simulink model "DFIG_BESS_In_power_LFnetwork_5bus"  (R2017b)
settings: Solver=ode23tb  StartTime=0.0  StopTime=7.5  MaxStep=0.04  RelTol=1e-3  EnableMultiTasking=on
values from neighbouring files (symbols this model uses):
  beta = beta (k)    [Parameter_2M_DFIG_BESS.m]
  Cbus = 80e-3    (= 0.08)    [Parameter_2M_DFIG_BESS.m]
  Cbus_bess = 15e-3    (= 0.015)    [Parameter_2M_DFIG_BESS.m]
  Cfilter = 80e-3    (= 0.08)    [Parameter_2M_DFIG_BESS.m]
  cp_opt_abs = abs(max(Cp))    [Parameter_2M_DFIG_BESS.m]
  D = 0.1    [Parameter_2M_DFIG_BESS.m]
  f = 60    [Parameter_2M_DFIG_BESS.m]
  Fs = 1.5    [Parameter_2M_DFIG_BESS.m]
  fsw = 4e3    (= 4000)    [Parameter_2M_DFIG_BESS.m]
  J = 90    [Parameter_2M_DFIG_BESS.m]
  ki_id = (wni^2)*Lr*sigma    (= 491.599501999)    [Parameter_2M_DFIG_BESS.m]
  ki_idg = (wnig^2)*Lg    (= 68.6450725305)    [Parameter_2M_DFIG_BESS.m]
  ki_iq = ki_id    (= 491.599501999)    [Parameter_2M_DFIG_BESS.m]
  ki_iqg = ki_idg    (= 68.6450725305)    [Parameter_2M_DFIG_BESS.m]
  ki_v = -300000    [Parameter_2M_DFIG_BESS.m]
  kp_id = (2*wni*sigma*Lr)-Rr    (= 0.5771)    [Parameter_2M_DFIG_BESS.m]
  kp_idg = (2*wnig*Lg)-Rg    (= 0.364153420404)    [Parameter_2M_DFIG_BESS.m]
  kp_iq = kp_id    (= 0.5771)    [Parameter_2M_DFIG_BESS.m]
  kp_iqg = kp_idg    (= 0.364153420404)    [Parameter_2M_DFIG_BESS.m]
  kp_v = -1000    [Parameter_2M_DFIG_BESS.m]
  Kpg = 1/(1.5*Vs*sqrt(2/3))    [Parameter_2M_DFIG_BESS.m]
  Kqg = -Kpg    [Parameter_2M_DFIG_BESS.m]
  lambda_opt = abs(lambda(posicion))    [Parameter_2M_DFIG_BESS.m]
  Lfilter = 483e-6    (= 0.000483)    [Parameter_2M_DFIG_BESS.m]
  Lg = 483e-6    (= 0.000483)    [Parameter_2M_DFIG_BESS.m]
  Lm = 2.5e-3    (= 0.0025)    [Parameter_2M_DFIG_BESS.m]
  Lr = Lm + Lsr    (= 0.002587)    [Parameter_2M_DFIG_BESS.m]
  Ls = Lm + Lsi    (= 0.002587)    [Parameter_2M_DFIG_BESS.m]
  Lsi = 87e-6    (= 8.7e-05)    [Parameter_2M_DFIG_BESS.m]
  n = 1800    [Parameter_2M_DFIG_BESS.m]
  N = 100    [Parameter_2M_DFIG_BESS.m]
  p = 2    [Parameter_2M_DFIG_BESS.m]
  Ps = 2e6    (= 2000000)    [Parameter_2M_DFIG_BESS.m]
  Radio = 44    [Parameter_2M_DFIG_BESS.m]
  Rfilter = 20e-3    (= 0.02)    [Parameter_2M_DFIG_BESS.m]
  ro = 1.225    [Parameter_2M_DFIG_BESS.m]
  Rr = 2.9e-3    (= 0.0029)    [Parameter_2M_DFIG_BESS.m]
  Rs = 2.6e-3    (= 0.0026)    [Parameter_2M_DFIG_BESS.m]
  sigma = 1- Lm^2/(Ls*Lr)    (= 0.0661284179513)    [Parameter_2M_DFIG_BESS.m]
  Ts = 1/fsw/f    (= 4.16666666667e-06)    [Parameter_2M_DFIG_BESS.m]
  Vbus_ref = 1200    [Parameter_2M_DFIG_BESS.m]
  Vdc_bat_ref = 1300    [Parameter_2M_DFIG_BESS.m]
  Vs = 690    [Parameter_2M_DFIG_BESS.m]
undefined symbols (not defined in the file or in its folder): D1, D11, Delta, DiscIntNeverNeededParam, Ion, Lithium, sigbuilder_block
libraries: powerlib x83, powerlib_meascontrol x28, sps_avr x2, electricdrivelib x1, peGeneralControl x1
(part 1 of 3)
Description:
  | Copyright 2008-2017 The MathWorks, Inc.
settings Model: Creator=MathWorks  LastModifiedBy=admin
settings DataIOCC: LimitDataPoints=on  SaveFormat=Array  SignalLoggingSaveFormat=ModelDataLogs
settings OptimizationCC: ExpressionDepthLimit=2147483647  LifeSpan=inf
settings DebuggingCC: UnderspecifiedInitializationDetection=Classic  MergeDetectMultiDrivingBlocksExec=none  MaxConsecutiveZCsMsg=none  SolverPrmCheckMsg=warning  FcnCallInpInsideContextMsg=warning  UnconnectedInputMsg=none  UnconnectedOutputMsg=none  UnconnectedLineMsg=none  StateNameClashWarn=warning  SFUnexpectedBacktrackingDiag=warning  SFNoUnconditionalDefaultTransitionDiag=warning  SFExecutionAtInitializationDiag=none
settings HardwareCC: ProdBitPerPointer=32  ProdBitPerSizeT=32  ProdBitPerPtrDiffT=32  ProdLargestAtomicFloat=None  ProdIntDivRoundTo=Undefined  ProdEndianess=Unspecified  ProdWordSize=32  ProdHWDeviceType=32-bit Generic
settings ModelReferenceCC: PropagateSignalLabelsOutOfModel=off
settings CodeAppCC: StateflowObjectComments=on
settings GRTTargetCC: TargetLangStandard=C89/C90 (ANSI)  GeneratePreprocessorConditionals=Disable all  CombineOutputUpdateFcns=off  GRTInterface=on
settings ConfigComp: CovMetricSettings=dw  CovHtmlReporting=on  CovSaveCumulativeToWorkspaceVar=on  CovSaveSingleToWorkspaceVar=on  CovExternalEMLEnable=off  CovSFcnEnable=off
settings SimscapeCC: SimscapeNormalizeSystem=off

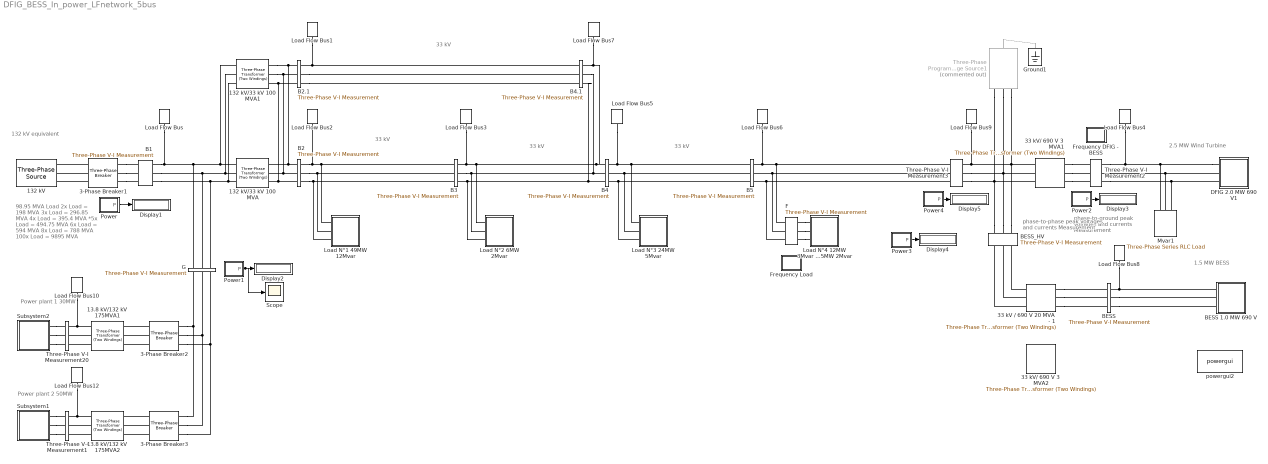
== system DFIG_BESS_In_power_LFnetwork_5bus ==
  note: 98.95 MVA Load
      | 2x Load = 198 MVA
      | 3x Load = 296.85 MVA
      | 4x Load = 395.4 MVA
      | *5x Load = 494.75 MVA
      | 6x Load = 594 MVA
      | 8x Load = 788 MVA
      | 100x Load = 9895 MVA
  note: 2.5 MW Wind Turbine
  note: 33 kV
  note: 132 kV equivalent
  note: 33 kV
  note: 33 kV
  note: phase-to-ground peak voltages
      | and currents Measurement
  note: 33 kV
  note: 1.5 MW BESS
  note: Power plant 1
      | 30MW
  note: Power plant 2
      | 50MW
  note: phase-to-phase peak voltages
      | and currents Measurement
  13.8 kV/132 kV 175MVA1 : powerlib/Elements/Three-Phase Transformer (Two Windings)  Winding1Connection=Delta (D1)  Winding2Connection=Yg  CoreType=Three single-phase transformers  SetSaturation=off  Hysteresis=off  DataFile='basic_model'  SetInitialFlux=off  Measurements=None  UNITS=pu  NominalPower=[100e6 60]  Winding1="[13.8e3  0.002   0.08 ]"  Winding2="[ 132e3  0.002  0.08]"  Rm=500  Lm=500  L0=0.5  Saturation="[ 0,0  ;  0.005,1.2  ;  1.0,1.4 ]"  InitialFluxes=[ 0.8 , -0.8 , 0.7 ]  MoreParameters=off  BreakLoop=off  DataType=off  TransfoNumber=0
  13.8 kV/132 kV 175MVA2 : powerlib/Elements/Three-Phase Transformer (Two Windings)  Winding1Connection=Delta (D1)  Winding2Connection=Yg  CoreType=Three single-phase transformers  SetSaturation=off  Hysteresis=off  DataFile='basic_model'  SetInitialFlux=off  Measurements=None  UNITS=pu  NominalPower=[100e6 60]  Winding1="[13.8e3  0.002   0.08 ]"  Winding2="[ 132e3  0.002  0.08]"  Rm=500  Lm=500  L0=0.5  Saturation="[ 0,0  ;  0.005,1.2  ;  1.0,1.4 ]"  InitialFluxes=[ 0.8 , -0.8 , 0.7 ]  MoreParameters=off  BreakLoop=off  DataType=off  TransfoNumber=0
  132 kV : powerlib/Electrical Sources/Three-Phase Source  InternalConnection=Yg  VoltagePhases=off  Voltage=(132000)  PhaseAngle=-3.3182  Voltage_phases=[25e3 25e3 25e3]/sqrt(3)  PhaseAngles_phases=[0 -120 +120]  Frequency=60  NonIdealSource=on  SpecifyImpedance=on  Resistance=0.8929  Inductance=16.58e-3  ShortCircuitLevel=494e6  BaseVoltage=120e3  XRratio=7  BusType=swing  Pref=10000000  Qref=3000000  Prefabc=[10e3, 10e3, 10e3]  Qrefabc=[0, 0, 0]  Qmin=-Inf  Qmax=Inf
  132 kV/33 kV 100 MVA : powerlib/Elements/Three-Phase Transformer (Two Windings)  Winding1Connection=Yg  Winding2Connection=Delta (D1)  CoreType=Three single-phase transformers  SetSaturation=off  Hysteresis=off  DataFile='basic_model'  SetInitialFlux=off  Measurements=None  UNITS=pu  NominalPower=[100e6 60 ]  Winding1="[ 132e3  0.002    0.06 ]"  Winding2="[ 33e3  0.002  0.06]"  Rm=500  Lm=500  L0=0.5  Saturation="[ 0,0  ;  0.005,1.2  ;  1.0,1.4 ]"  InitialFluxes=[ 0.8 , -0.8 , 0.7 ]  MoreParameters=off  BreakLoop=off  DataType=off  TransfoNumber=0
  132 kV/33 kV 100 MVA1 : powerlib/Elements/Three-Phase Transformer (Two Windings)  Winding1Connection=Yg  Winding2Connection=Delta (D1)  CoreType=Three single-phase transformers  SetSaturation=off  Hysteresis=off  DataFile='basic_model'  SetInitialFlux=off  Measurements=None  UNITS=pu  NominalPower=[100e6 60 ]  Winding1="[ 132e3  0.002    0.06 ]"  Winding2="[ 33e3  0.002  0.06]"  Rm=500  Lm=500  L0=0.5  Saturation="[ 0,0  ;  0.005,1.2  ;  1.0,1.4 ]"  InitialFluxes=[ 0.8 , -0.8 , 0.7 ]  MoreParameters=off  BreakLoop=off  DataType=off  TransfoNumber=0
  3-Phase Breaker1 : powerlib/Elements/Three-Phase Breaker  InitialState=closed  SwitchA=on  SwitchB=on  SwitchC=on  SwitchTimes=[5]  External=off  BreakerResistance=0.001  SnubberResistance=1e6  SnubberCapacitance=inf  Measurements=None
      settings: AttributesFormatString=\n
  3-Phase Breaker2 : powerlib/Elements/Three-Phase Breaker  InitialState=closed  SwitchA=on  SwitchB=on  SwitchC=on  SwitchTimes=[105.025]  External=off  BreakerResistance=0.001  SnubberResistance=1e6  SnubberCapacitance=inf  Measurements=None
      settings: AttributesFormatString=\n
  3-Phase Breaker3 : powerlib/Elements/Three-Phase Breaker  InitialState=closed  SwitchA=on  SwitchB=on  SwitchC=on  SwitchTimes=[105.0]  External=off  BreakerResistance=0.001  SnubberResistance=1e6  SnubberCapacitance=inf  Measurements=None
      settings: AttributesFormatString=\n
  33 kV / 690 V 20 MVA - 1 : powerlib/Elements/Three-Phase Transformer (Two Windings)  Winding1Connection=Delta (D11)  Winding2Connection=Yg  CoreType=Three single-phase transformers  SetSaturation=off  Hysteresis=off  DataFile='hysteresis'  SetInitialFlux=off  Measurements=None  UNITS=SI  NominalPower="[2e6  f]"  Winding1=[33000 0.14881 0.011842]  Winding2=[690 200e-3 2.0881e-06]  Rm=89286  Lm=Inf  L0=0.5  Saturation=[0 0;0.47518 112.54;197.99 142.55]  InitialFluxes=[75.026 -75.026 65.648]  MoreParameters=off  BreakLoop=off  DataType=on  TransfoNumber=0
  33 kV/ 690 V 3 MVA1 : powerlib/Elements/Three-Phase Transformer (Two Windings)  Winding1Connection=Yg  Winding2Connection=Yg  CoreType=Three single-phase transformers  SetSaturation=off  Hysteresis=off  DataFile='hysteresis'  SetInitialFlux=off  Measurements=None  UNITS=pu  NominalPower="[3e6  f]"  Winding1=[33e3 , 0.025/30 , 0.025]  Winding2=[ 690, 0.025/30 , 0.025]  Rm=89286  Lm=inf  L0=0.5  Saturation=[ 0,0 ; 0.0024,1.2 ; 1.0,1.52 ]  InitialFluxes=[ 0.8 , -0.8 , 0.7 ]  MoreParameters=off  BreakLoop=off  DataType=off  TransfoNumber=0
  33 kV/ 690 V 3 MVA2 : powerlib/Elements/Three-Phase Transformer (Two Windings)  Winding1Connection=Yg  Winding2Connection=Yg  CoreType=Three single-phase transformers  SetSaturation=off  Hysteresis=off  DataFile='hysteresis'  SetInitialFlux=off  Measurements=None  UNITS=pu  NominalPower="[2e6  f]"  Winding1=[33e3 , 0.025/30 , 0.025]  Winding2=[ 690, 0.025/30 , 0.025]  Rm=89286  Lm=inf  L0=0.5  Saturation=[ 0,0 ; 0.0024,1.2 ; 1.0,1.52 ]  InitialFluxes=[ 0.8 , -0.8 , 0.7 ]  MoreParameters=off  BreakLoop=off  DataType=off  TransfoNumber=0
  B1 : powerlib/Measurements/Three-Phase V-I Measurement  VoltageMeasurement=phase-to-phase  SetLabelV=on  LabelV=Vabc_B1  Vpu=off  VpuLL=off  CurrentMeasurement=yes  SetLabelI=on  LabelI=Iabc_B1  Ipu=off  Pbase=100e6  Vbase=132e3  OutputType=Complex  PhasorSimulation=off  PSBequivalent=0
  B2 : powerlib/Measurements/Three-Phase V-I Measurement  VoltageMeasurement=no  SetLabelV=off  LabelV=Vabc_B2  Vpu=off  VpuLL=off  CurrentMeasurement=no  SetLabelI=on  LabelI=Iabc_B120  Ipu=off  Pbase=100e6  Vbase=33e3  OutputType=Complex  PhasorSimulation=off  PSBequivalent=0
  B2.1 : powerlib/Measurements/Three-Phase V-I Measurement  VoltageMeasurement=no  SetLabelV=on  LabelV=Vabc_B2  Vpu=on  VpuLL=off  CurrentMeasurement=no  SetLabelI=on  LabelI=Iabc_B120  Ipu=off  Pbase=100e6  Vbase=33e3  OutputType=Complex  PhasorSimulation=off  PSBequivalent=0
  B3 : powerlib/Measurements/Three-Phase V-I Measurement  VoltageMeasurement=no  SetLabelV=on  LabelV=Vabc_B3  Vpu=on  VpuLL=off  CurrentMeasurement=no  SetLabelI=on  LabelI=Iabc_B120  Ipu=off  Pbase=100e6  Vbase=33e3  OutputType=Complex  PhasorSimulation=off  PSBequivalent=0
  B4 : powerlib/Measurements/Three-Phase V-I Measurement  VoltageMeasurement=no  SetLabelV=on  LabelV=Vabc_B4  Vpu=on  VpuLL=off  CurrentMeasurement=no  SetLabelI=on  LabelI=Iabc_B120  Ipu=off  Pbase=100e6  Vbase=33e3  OutputType=Complex  PhasorSimulation=off  PSBequivalent=0
  B4.1 : powerlib/Measurements/Three-Phase V-I Measurement  VoltageMeasurement=no  SetLabelV=on  LabelV=Vabc_B4  Vpu=on  VpuLL=off  CurrentMeasurement=no  SetLabelI=on  LabelI=Iabc_B120  Ipu=off  Pbase=100e6  Vbase=33e3  OutputType=Complex  PhasorSimulation=off  PSBequivalent=0
  B5 : powerlib/Measurements/Three-Phase V-I Measurement  VoltageMeasurement=no  SetLabelV=on  LabelV=Vabc_B5  Vpu=on  VpuLL=off  CurrentMeasurement=no  SetLabelI=on  LabelI=Iabc_B120  Ipu=off  Pbase=100e6  Vbase=33e3  OutputType=Complex  PhasorSimulation=off  PSBequivalent=0
  BESS : powerlib/Measurements/Three-Phase V-I Measurement  VoltageMeasurement=phase-to-phase  SetLabelV=on  LabelV=V_ac_bat_low  Vpu=off  VpuLL=off  CurrentMeasurement=yes  SetLabelI=on  LabelI=I_ac_bat_low  Ipu=off  Pbase=100e6  Vbase=500e3  OutputType=Complex  PhasorSimulation=off  PSBequivalent=0
  BESS 1.0 MW 690 V : Subsystem
  BESS_HV : powerlib/Measurements/Three-Phase V-I Measurement  VoltageMeasurement=phase-to-phase  SetLabelV=on  LabelV=V_ac_bess_HV  Vpu=off  VpuLL=off  CurrentMeasurement=yes  SetLabelI=on  LabelI=I_ac_bess_HV  Ipu=off  Pbase=100e6  Vbase=500e3  OutputType=Complex  PhasorSimulation=off  PSBequivalent=0
  DFIG 2.0 MW 690 V1 : Subsystem
  Display{1..5} (5 alike) : Display
  F : powerlib/Measurements/Three-Phase V-I Measurement  VoltageMeasurement=phase-to-ground  SetLabelV=on  LabelV=Vabc_h_plant  Vpu=off  VpuLL=off  CurrentMeasurement=no  SetLabelI=on  LabelI=Iabc_B120  Ipu=off  Pbase=100e6  Vbase=120e3  OutputType=Complex  PhasorSimulation=off  PSBequivalent=0
  Frequency Load : Subsystem
  Frequency DFIG - BESS : Subsystem
  G : powerlib/Measurements/Three-Phase V-I Measurement  VoltageMeasurement=phase-to-phase  SetLabelV=on  LabelV=Vabc_G  Vpu=off  VpuLL=off  CurrentMeasurement=yes  SetLabelI=on  LabelI=Iabc_G  Ipu=off  Pbase=100e6  Vbase=132e3  OutputType=Complex  PhasorSimulation=off  PSBequivalent=0
  Ground1 : powerlib/Elements/Ground  LConnTagsString=a
  Load Flow Bus : powerlib/Measurements/Load Flow Bus  LConnTagsString=a  Phases=single  Connectors=on one side  ID=B1  Vbase=132e3  Vref=1.02  Vangle=0  VLF=1.02  VLFb=1  VLFc=1  angleLF=0  angleLFb=0  angleLFc=0
      settings: AttributesFormatString=%<ID>\n%<Vbase>V\n%<VLF>pu\n%<angleLF>deg.  SourceProductName=Simscape Power Systems
  Load Flow Bus1 : powerlib/Measurements/Load Flow Bus  LConnTagsString=a  Phases=single  Connectors=on one side  ID=B2.1  Vbase=33e3  Vref=1  Vangle=0  VLF=0.9983  VLFb=1  VLFc=1  angleLF=-30.23  angleLFb=0  angleLFc=0
      settings: AttributesFormatString=%<ID>\n%<Vbase>V\n%<VLF>pu\n%<angleLF>deg.  SourceProductName=Simscape Power Systems
  Load Flow Bus10 : powerlib/Measurements/Load Flow Bus  LConnTagsString=a  Phases=single  Connectors=on one side  ID=B13.8  Vbase=13.8e3  Vref=0.98  Vangle=0  VLF=0.98  VLFb=1  VLFc=1  angleLF=-23.81  angleLFb=0  angleLFc=0
      settings: AttributesFormatString=%<ID>\n%<Vbase>V\n%<VLF>pu\n%<angleLF>deg.  SourceProductName=Simscape Power Systems
  Load Flow Bus12 : powerlib/Measurements/Load Flow Bus  LConnTagsString=a  Phases=single  Connectors=on one side  ID=B13.8  Vbase=13.8e3  Vref=0.98  Vangle=0  VLF=0.98  VLFb=1  VLFc=1  angleLF=-23.81  angleLFb=0  angleLFc=0
      settings: AttributesFormatString=%<ID>\n%<Vbase>V\n%<VLF>pu\n%<angleLF>deg.  SourceProductName=Simscape Power Systems
  Load Flow Bus2 : powerlib/Measurements/Load Flow Bus  LConnTagsString=a  Phases=single  Connectors=on one side  ID=B2  Vbase=33e3  Vref=1  Vangle=0  VLF=0.9983  VLFb=1  VLFc=1  angleLF=-30.23  angleLFb=0  angleLFc=0
      settings: AttributesFormatString=%<ID>\n%<Vbase>V\n%<VLF>pu\n%<angleLF>deg.  SourceProductName=Simscape Power Systems
  Load Flow Bus3 : powerlib/Measurements/Load Flow Bus  LConnTagsString=a  Phases=single  Connectors=on one side  ID=B3  Vbase=33e3  Vref=1  Vangle=0  VLF=0.9671  VLFb=1  VLFc=1  angleLF=-20.87  angleLFb=0  angleLFc=0
      settings: AttributesFormatString=%<ID>\n%<Vbase>V\n%<VLF>pu\n%<angleLF>deg.  SourceProductName=Simscape Power Systems
  Load Flow Bus4 : powerlib/Measurements/Load Flow Bus  LConnTagsString=a  Phases=single  Connectors=on one side  ID=B690  Vbase=690  Vref=1  Vangle=0  VLF=0.9532  VLFb=1  VLFc=1  angleLF=-18.54  angleLFb=0  angleLFc=0
      settings: AttributesFormatString=%<ID>\n%<Vbase>V\n%<VLF>pu\n%<angleLF>deg.  SourceProductName=Simscape Power Systems
  Load Flow Bus5 : powerlib/Measurements/Load Flow Bus  LConnTagsString=a  Phases=single  Connectors=on one side  ID=B4  Vbase=33e3  Vref=1  Vangle=0  VLF=0.9671  VLFb=1  VLFc=1  angleLF=-20.87  angleLFb=0  angleLFc=0
      settings: AttributesFormatString=%<ID>\n%<Vbase>V\n%<VLF>pu\n%<angleLF>deg.  SourceProductName=Simscape Power Systems
  Load Flow Bus6 : powerlib/Measurements/Load Flow Bus  LConnTagsString=a  Phases=single  Connectors=on one side  ID=B5  Vbase=33e3  Vref=1  Vangle=0  VLF=0.9671  VLFb=1  VLFc=1  angleLF=-20.87  angleLFb=0  angleLFc=0
      settings: AttributesFormatString=%<ID>\n%<Vbase>V\n%<VLF>pu\n%<angleLF>deg.  SourceProductName=Simscape Power Systems
  Load Flow Bus7 : powerlib/Measurements/Load Flow Bus  LConnTagsString=a  Phases=single  Connectors=on one side  ID=B4.1  Vbase=33e3  Vref=1  Vangle=0  VLF=0.9671  VLFb=1  VLFc=1  angleLF=-20.87  angleLFb=0  angleLFc=0
      settings: AttributesFormatString=%<ID>\n%<Vbase>V\n%<VLF>pu\n%<angleLF>deg.  SourceProductName=Simscape Power Systems
  Load Flow Bus8 : powerlib/Measurements/Load Flow Bus  LConnTagsString=a  Phases=single  Connectors=on one side  ID=B690_BESS  Vbase=690  Vref=1  Vangle=0  VLF=0.9532  VLFb=1  VLFc=1  angleLF=-18.54  angleLFb=0  angleLFc=0
      settings: AttributesFormatString=%<ID>\n%<Vbase>V\n%<VLF>pu\n%<angleLF>deg.  SourceProductName=Simscape Power Systems
  Load Flow Bus9 : powerlib/Measurements/Load Flow Bus  LConnTagsString=a  Phases=single  Connectors=on one side  ID=B6  Vbase=33e3  Vref=1  Vangle=0  VLF=0.9671  VLFb=1  VLFc=1  angleLF=-20.87  angleLFb=0  angleLFc=0
      settings: AttributesFormatString=%<ID>\n%<Vbase>V\n%<VLF>pu\n%<angleLF>deg.  SourceProductName=Simscape Power Systems
  Load N°1 49MW 12Mvar : Subsystem
  Load N°2 6MW 2Mvar : Subsystem
  Load N°3 24MW 5Mvar : Subsystem
  Load N°4 12MW 3Mvar Load N°5 5MW 2Mvar : Subsystem
  Mvar1 : powerlib/Elements/Three-Phase Series RLC Load  LConnTagsString=A|B|C  Configuration=Delta  NominalVoltage=575  Vabc=[1e3 1e3 1e3]  Vabcp=[1e3 1e3 1e3]  NominalFrequency=60  UnbalancedPower=off  ActivePower=0.05e6/50  InductivePower=0  CapacitivePower=0.05e6  Pabc=[10e3 9e3 11e3]  QLabc=[100 90 110]  QCabc=[100 90 110]  Pabcp=[10e3 9e3 11e3]  QLabcp=[100 90 110]  QCabcp=[100 90 110]  Measurements=None  LoadType=constant Z
  Power : Subsystem
  Power1 : Subsystem
  Power2 : Subsystem
  Power3 : Subsystem
  Power4 : Subsystem
  Scope : Scope
  Subsystem1 : Subsystem
  Subsystem2 : Subsystem
  Three-Phase Programmable Voltage Source1 : powerlib/Electrical Sources/Three-Phase Programmable Voltage Source  Commented=on  PositiveSequence="[33e3  0 f]"  VariationEntity=None  VariationType=Table of time-amplitude pairs  VariationTypeAlt=Step  VariationStep=[-0.5]  VariationRate=-0.3  VariationMagnitude=0.3  VariationFrequency=2  VariationTiming=[5 7.5]  VariationPhaseA=off  Amplitudes=[1 0.95 1]  TimeValues=[0 0.9 2]  HarmonicGeneration=off  HarmonicA=[3 0.2 -25 0]  HarmonicB=[2 0.15 35 2]  Timing="[0.05  3]"  BusType=swing  Pref=0  Qref=0  Qmin=-inf  Qmax=inf
  Three-Phase V-I Measurement1 : powerlib/Measurements/Three-Phase V-I Measurement  VoltageMeasurement=no  SetLabelV=off  LabelV=V_ac_syn_low_2  Vpu=off  VpuLL=off  CurrentMeasurement=no  SetLabelI=off  LabelI=I_ac_syn_low_2  Ipu=off  Pbase=100e6  Vbase=500e3  OutputType=Complex  PhasorSimulation=off  PSBequivalent=0
  Three-Phase V-I Measurement2 : powerlib/Measurements/Three-Phase V-I Measurement  VoltageMeasurement=phase-to-ground  SetLabelV=on  LabelV=V_ac_g  Vpu=off  VpuLL=off  CurrentMeasurement=yes  SetLabelI=on  LabelI=I_ac_g  Ipu=off  Pbase=100e6  Vbase=500e3  OutputType=Complex  PhasorSimulation=off  PSBequivalent=0
  Three-Phase V-I Measurement20 : powerlib/Measurements/Three-Phase V-I Measurement  VoltageMeasurement=no  SetLabelV=on  LabelV=V_ac_syn_low  Vpu=off  VpuLL=off  CurrentMeasurement=no  SetLabelI=on  LabelI=I_ac_syn_low  Ipu=off  Pbase=100e6  Vbase=500e3  OutputType=Complex  PhasorSimulation=off  PSBequivalent=0
  Three-Phase V-I Measurement3 : powerlib/Measurements/Three-Phase V-I Measurement  VoltageMeasurement=phase-to-ground  SetLabelV=on  LabelV=V_ac_g_Total  Vpu=off  VpuLL=off  CurrentMeasurement=yes  SetLabelI=on  LabelI=I_ac_g_Total  Ipu=off  Pbase=100e6  Vbase=500e3  OutputType=Complex  PhasorSimulation=off  PSBequivalent=0
  powergui2 : powerlib/powergui  Priority=1  SimulationMode=Discrete  SampleTime=Ts  frequency=60  Iterations=50  frequencyindice=0  Pbase=100e6  ErrMax=0.0001  UnitsV=kV  UnitsW=MW  buscounter=0  FunctionMessages=off  echomessages=off  EnableUseOfTLC=off  CurrentSourceSwitches=off  DisableSnubberDevices=off  DisableRonSwitches=off  DisableVfSwitches=off  DisplayEquations=off  SolverType=Tustin  Interpol=off  ExternalGateDelay=off  methode=off  Ts=100  x0status=blocks  SPID=off  SwTol=0  HookPort=off  RestoreLinks=warning  ResistiveCurrentMeasurement=off  Frange=[0:2:500]  Ylog=off  Xlog=on  ShowGrid=off  save=off  variable=ZData  structure=0  ZoomFFT=off  StartTime=0.0  cycles=1  DisplayStyle=1  fundamental=60  FreqAxis=off  MaxFrequency=1000  frequencyindicesteady=1  RmsSteady=1  display=off
  wires:
  Power/1(P) -> Display1/1
  Power1/1(P) -> Scope/1, Display2/1
  Power3/1(P) -> Display4/1
  Power2/1(P) -> Display3/1
  Power4/1(P) -> Display5/1
  connections:
  B2/LConn2 -- B2.1/LConn2 -- 132 kV/33 kV 100 MVA1/RConn2 -- 132 kV/33 kV 100 MVA/RConn2
  B2/LConn3 -- B2.1/LConn3 -- 132 kV/33 kV 100 MVA1/RConn3 -- 132 kV/33 kV 100 MVA/RConn3
  B1/RConn1 -- Load Flow Bus/LConn1 -- G/RConn1 -- 132 kV/33 kV 100 MVA1/LConn1 -- 132 kV/33 kV 100 MVA/LConn1
  B2/RConn3 -- B3/LConn3 -- Load N°1 49MW 12Mvar/RConn3
  Load Flow Bus2/LConn1 -- B2/RConn1 -- B3/LConn1 -- Load N°1 49MW 12Mvar/RConn1
  B1/RConn3 -- G/RConn3 -- 132 kV/33 kV 100 MVA1/LConn3 -- 132 kV/33 kV 100 MVA/LConn3
  B2/RConn2 -- B3/LConn2 -- Load N°1 49MW 12Mvar/RConn2
  B1/RConn2 -- G/RConn2 -- 132 kV/33 kV 100 MVA1/LConn2 -- 132 kV/33 kV 100 MVA/LConn2
  DFIG 2.0 MW 690 V1/RConn1 -- Mvar1/LConn1 -- Three-Phase V-I Measurement2/LConn1 -- Load Flow Bus4/LConn1
  Three-Phase V-I Measurement2/LConn2 -- Mvar1/LConn2 -- DFIG 2.0 MW 690 V1/RConn2
  Three-Phase V-I Measurement2/LConn3 -- Mvar1/LConn3 -- DFIG 2.0 MW 690 V1/RConn3
  B2/LConn1 -- B2.1/LConn1 -- 132 kV/33 kV 100 MVA1/RConn1 -- 132 kV/33 kV 100 MVA/RConn1
  B3/RConn2 -- B4.1/RConn2 -- B4/LConn2 -- Load N°2 6MW 2Mvar/RConn2
  B3/RConn3 -- B4.1/RConn3 -- B4/LConn3 -- Load N°2 6MW 2Mvar/RConn3
  Load Flow Bus3/LConn1 -- B3/RConn1 -- Load Flow Bus7/LConn1 -- B4.1/RConn1 -- B4/LConn1 -- Load N°2 6MW 2Mvar/RConn1
  Load N°3 24MW 5Mvar/RConn3 -- B5/LConn3 -- B4/RConn3
  Load Flow Bus5/LConn1 -- B4/RConn1 -- B5/LConn1 -- Load N°3 24MW 5Mvar/RConn1
  Load N°3 24MW 5Mvar/RConn2 -- B5/LConn2 -- B4/RConn2
  3-Phase Breaker1/LConn1 -- 132 kV/RConn1
  3-Phase Breaker1/LConn2 -- 132 kV/RConn2
  3-Phase Breaker1/LConn3 -- 132 kV/RConn3
  33 kV / 690 V 20 MVA - 1/RConn1 -- BESS/RConn1
  33 kV / 690 V 20 MVA - 1/RConn2 -- BESS/RConn2
  33 kV / 690 V 20 MVA - 1/RConn3 -- BESS/RConn3
  BESS/LConn1 -- Load Flow Bus8/LConn1 -- BESS 1.0 MW 690 V/RConn1
  BESS/LConn2 -- BESS 1.0 MW 690 V/RConn2
  BESS/LConn3 -- BESS 1.0 MW 690 V/RConn3
  B2.1/RConn1 -- B4.1/LConn1 -- Load Flow Bus1/LConn1
  B2.1/RConn2 -- B4.1/LConn2
  B2.1/RConn3 -- B4.1/LConn3
  Load Flow Bus6/LConn1 -- Three-Phase V-I Measurement3/RConn1 -- F/LConn1 -- B5/RConn1
  3-Phase Breaker1/RConn1 -- B1/LConn1
  3-Phase Breaker1/RConn2 -- B1/LConn2
  3-Phase Breaker1/RConn3 -- B1/LConn3
  F/RConn1 -- Load N°4 12MW 3Mvar Load N°5 5MW 2Mvar/RConn1
  F/RConn2 -- Load N°4 12MW 3Mvar Load N°5 5MW 2Mvar/RConn2
  F/RConn3 -- Load N°4 12MW 3Mvar Load N°5 5MW 2Mvar/RConn3
  Subsystem2/LConn2 -- Three-Phase V-I Measurement20/LConn2
  13.8 kV/132 kV 175MVA1/LConn2 -- Three-Phase V-I Measurement20/RConn2
  13.8 kV/132 kV 175MVA1/LConn3 -- Three-Phase V-I Measurement20/RConn3
  Subsystem2/LConn3 -- Three-Phase V-I Measurement20/LConn3
  Subsystem2/LConn1 -- Three-Phase V-I Measurement20/LConn1
  13.8 kV/132 kV 175MVA1/LConn1 -- Load Flow Bus10/LConn1 -- Three-Phase V-I Measurement20/RConn1
  3-Phase Breaker2/LConn1 -- 13.8 kV/132 kV 175MVA1/RConn1
  3-Phase Breaker2/LConn2 -- 13.8 kV/132 kV 175MVA1/RConn2
  3-Phase Breaker2/LConn3 -- 13.8 kV/132 kV 175MVA1/RConn3
  Load Flow Bus12/LConn1 -- 13.8 kV/132 kV 175MVA2/LConn1 -- Three-Phase V-I Measurement1/RConn1
  Subsystem1/LConn1 -- Three-Phase V-I Measurement1/LConn1
  Subsystem1/LConn3 -- Three-Phase V-I Measurement1/LConn3
  3-Phase Breaker3/LConn3 -- 13.8 kV/132 kV 175MVA2/RConn3
  13.8 kV/132 kV 175MVA2/LConn3 -- Three-Phase V-I Measurement1/RConn3
  13.8 kV/132 kV 175MVA2/LConn2 -- Three-Phase V-I Measurement1/RConn2
  3-Phase Breaker3/LConn2 -- 13.8 kV/132 kV 175MVA2/RConn2
  Subsystem1/LConn2 -- Three-Phase V-I Measurement1/LConn2
  3-Phase Breaker3/LConn1 -- 13.8 kV/132 kV 175MVA2/RConn1
  3-Phase Breaker2/RConn1 -- 3-Phase Breaker3/RConn1 -- G/LConn1
  3-Phase Breaker2/RConn2 -- 3-Phase Breaker3/RConn2 -- G/LConn2
  3-Phase Breaker2/RConn3 -- G/LConn3 -- 3-Phase Breaker3/RConn3
  33 kV / 690 V 20 MVA - 1/LConn1 -- BESS_HV/LConn1
  33 kV / 690 V 20 MVA - 1/LConn2 -- BESS_HV/LConn2
  33 kV / 690 V 20 MVA - 1/LConn3 -- BESS_HV/LConn3
  F/LConn2 -- B5/RConn2 -- Three-Phase V-I Measurement3/RConn2
  F/LConn3 -- B5/RConn3 -- Three-Phase V-I Measurement3/RConn3
  33 kV/ 690 V 3 MVA1/RConn1 -- Three-Phase V-I Measurement2/RConn1
  33 kV/ 690 V 3 MVA1/RConn2 -- Three-Phase V-I Measurement2/RConn2
  33 kV/ 690 V 3 MVA1/RConn3 -- Three-Phase V-I Measurement2/RConn3
  BESS_HV/RConn3 -- Three-Phase Programmable Voltage Source1/RConn3 -- 33 kV/ 690 V 3 MVA1/LConn3 -- Three-Phase V-I Measurement3/LConn3
  BESS_HV/RConn2 -- Three-Phase Programmable Voltage Source1/RConn2 -- 33 kV/ 690 V 3 MVA1/LConn2 -- Three-Phase V-I Measurement3/LConn2
  BESS_HV/RConn1 -- Three-Phase Programmable Voltage Source1/RConn1 -- Load Flow Bus9/LConn1 -- Three-Phase V-I Measurement3/LConn1 -- 33 kV/ 690 V 3 MVA1/LConn1
  Three-Phase Programmable Voltage Source1/LConn1 -- Ground1/LConn1

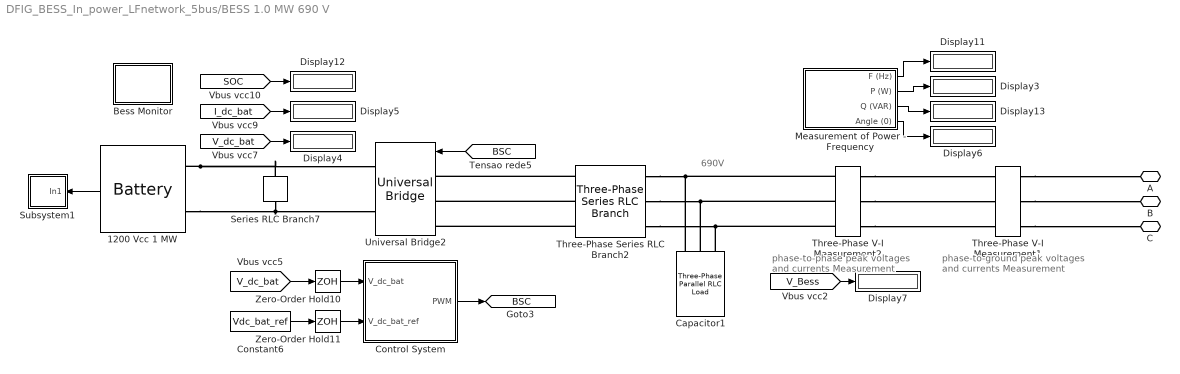
== system DFIG_BESS_In_power_LFnetwork_5bus/BESS 1.0 MW 690 V ==
  note: 690V
  note: phase-to-phase peak voltages
      | and currents Measurement
  note: phase-to-ground peak voltages
      | and currents Measurement
  "1200 Vcc 1 MW " : electricdrivelib/Extra Sources/Battery  BatType=Lithium-Ion  ShowTempParam=off  ThermalPreset=no  ShowAgeParam=off  NomV=1200  NomQ=1250  SOC=71  Batt_Tr=30  PresetModel=on  MaxQ=1250  MinV=900  FullV=1396.7846  Dis_rate=543.4783  R=0.0096  Normal_OP=1130.4348  expZone="[1296.463      61.413043]"  current=[833]  Units=Time  Tci=20  NomT=25  T2=0  MaxQ2=2.208  FullV2=3.45  Normal_OP2=2.8  expZone2="[3.22        0.23]"  Rca=0.6  ti=1000  Dp=0  Neq0=0  Tsim=1e6  Ta1=25  Qeol=5.4*0.9  Reol=0.013333*1.2  Char_age=[2.3478, 3]  Dis_age=[2.3478, 10]  N1=1500  N2=10500  N3=1000  N4=1400  Ta2=45  N5=950
  Bess Monitor : Subsystem
  Capacitor1 : powerlib/Elements/Three-Phase Parallel RLC Load  LConnTagsString=A|B|C  Configuration=Y (grounded)  NominalVoltage=Vs  Vabc=[1e3 1e3 1e3]  Vabcp=[1e3 1e3 1e3]  NominalFrequency=f  UnbalancedPower=off  ActivePower=0  InductivePower=0  CapacitivePower=Cfilter*2.5  Pabc=[10e3 9e3 11e3]  QLabc=[100 90 110]  QCabc=[100 90 110]  Pabcp=[10e3 9e3 11e3]  QLabcp=[100 90 110]  QCabcp=[100 90 110]  Measurements=None  LoadType=constant Z
  Constant6 : Constant  Value=Vdc_bat_ref
  Control System : Subsystem
  Display{3..7,11..13} (8 alike) : Display
  Measurement of Power - Frequency : Subsystem
  Series RLC Branch7 : powerlib/Elements/Series RLC Branch  LConnTagsString=__new0  RConnTagsString=__new0  BranchType=C  Resistance=1  Inductance=1e-3  SetiL0=off  InitialCurrent=0  Capacitance=Cbus_bess  Setx0=off  InitialVoltage=0  Measurements=Branch voltage
  Subsystem1 : Subsystem
  Three-Phase Series RLC Branch2 : powerlib/Elements/Three-Phase Series RLC Branch  LConnTagsString=A|B|C  RConnTagsString=A|B|C  BranchType=RL  Resistance=Rfilter  Inductance=Lfilter*1.5  Capacitance=0  Measurements=None
  Three-Phase V-I Measurement1 : powerlib/Measurements/Three-Phase V-I Measurement  VoltageMeasurement=phase-to-ground  SetLabelV=on  LabelV=V_ac_bess_2  Vpu=off  VpuLL=off  CurrentMeasurement=yes  SetLabelI=on  LabelI=I_ac_bess_2  Ipu=off  Pbase=100e6  Vbase=Vs  OutputType=Complex  PhasorSimulation=off  PSBequivalent=0
  Three-Phase V-I Measurement2 : powerlib/Measurements/Three-Phase V-I Measurement  VoltageMeasurement=phase-to-phase  SetLabelV=on  LabelV=V_ac_bess  Vpu=off  VpuLL=off  CurrentMeasurement=yes  SetLabelI=on  LabelI=I_ac_bess  Ipu=off  Pbase=100e6  Vbase=Vs  OutputType=Complex  PhasorSimulation=off  PSBequivalent=0
  Universal Bridge2 : powerlib/Power Electronics/Universal Bridge  Arms=3  SnubberResistance=1e5  SnubberCapacitance=inf  Device=Ideal Switches  Ron=1e-3  Lon=0  ForwardVoltages="[  0  0  ]"  ForwardVoltage=0  GTOparameters=[ 10e-6 , 20e-6 ]  IGBTparameters=[ 1e-6 , 2e-6 ]  Measurements=None  Measurements_2=None  converterType=Rectifier
  Zero-Order Hold10 : ZeroOrderHold  SampleTime=1/fsw
  Zero-Order Hold11 : ZeroOrderHold  SampleTime=1/fsw
  A : PMIOPort  Port=1  Side=Right
  B : PMIOPort  Port=2  Side=Right
  C : PMIOPort  Port=3  Side=Right
  tag scope: BSC=global
  wires:
  Zero-Order Hold10/1 -> Control System/1(V_dc_bat)
  [V_dc_bat] -> Zero-Order Hold10/1
  [I_dc_bat] -> Display5/1
  Control System/1(PWM) -> [BSC]
  Zero-Order Hold11/1 -> Control System/2(V_dc_bat_ref)
  [V_dc_bat] -> Display4/1
  "1200 Vcc 1 MW "/1 -> Subsystem1/1(In1)
  Constant6/1 -> Zero-Order Hold11/1
  [BSC] -> Universal Bridge2/1
  Measurement of Power - Frequency/2(P (W)) -> Display3/1
  Measurement of Power - Frequency/1(F (Hz)) -> Display11/1
  Measurement of Power - Frequency/3(Q (VAR)) -> Display13/1
  [SOC] -> Display12/1
  Measurement of Power - Frequency/4(Angle (0)) -> Display6/1
  [V_Bess] -> Display7/1
  connections:
  Series RLC Branch7/RConn1 -- "1200 Vcc 1 MW "/LConn2 -- Universal Bridge2/RConn2
  "1200 Vcc 1 MW "/LConn1 -- Series RLC Branch7/LConn1 -- Universal Bridge2/RConn1
  Three-Phase V-I Measurement2/LConn1 -- Capacitor1/LConn1 -- Three-Phase Series RLC Branch2/RConn1
  Three-Phase V-I Measurement2/LConn2 -- Capacitor1/LConn2 -- Three-Phase Series RLC Branch2/RConn2
  Three-Phase V-I Measurement2/LConn3 -- Capacitor1/LConn3 -- Three-Phase Series RLC Branch2/RConn3
  Three-Phase Series RLC Branch2/LConn1 -- Universal Bridge2/LConn1
  Three-Phase Series RLC Branch2/LConn2 -- Universal Bridge2/LConn2
  Three-Phase Series RLC Branch2/LConn3 -- Universal Bridge2/LConn3
  Three-Phase V-I Measurement2/RConn1 -- Three-Phase V-I Measurement1/LConn1
  Three-Phase V-I Measurement2/RConn2 -- Three-Phase V-I Measurement1/LConn2
  Three-Phase V-I Measurement2/RConn3 -- Three-Phase V-I Measurement1/LConn3
  Three-Phase V-I Measurement1/RConn1 -- A/RConn1
  Three-Phase V-I Measurement1/RConn2 -- B/RConn1
  Three-Phase V-I Measurement1/RConn3 -- C/RConn1

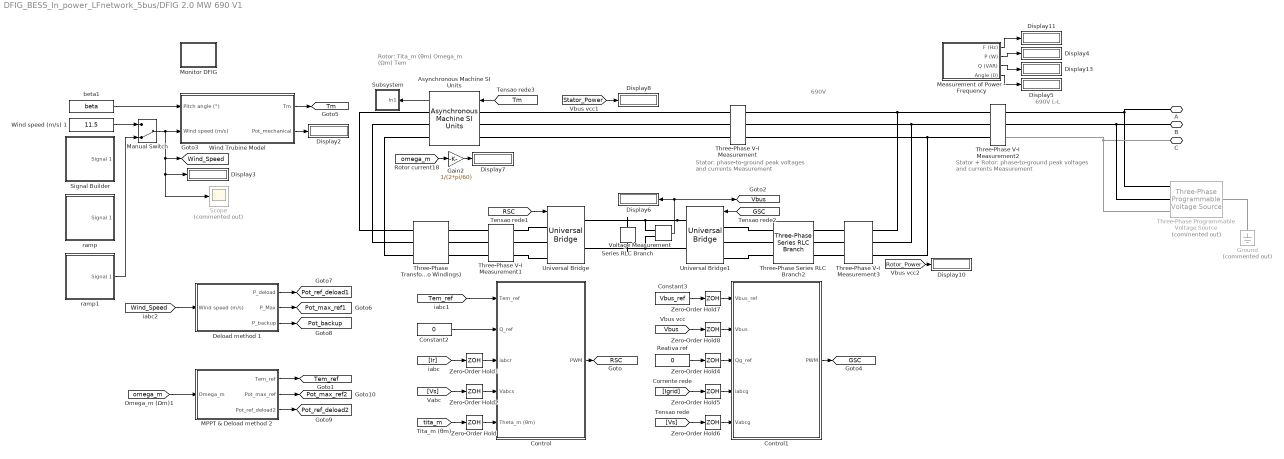
== system DFIG_BESS_In_power_LFnetwork_5bus/DFIG 2.0 MW 690 V1 ==
  note: 690V L-L
  note: Rotor:
      | Tita_m (θm)
      | Omega_m (Ωm)
      | Tem
  note: 690V
  note: Stator + Rotor: phase-to-ground peak voltages
      | and currents Measurement
  note: Stator: phase-to-ground peak voltages
      | and currents Measurement
  Asynchronous Machine SI Units : powerlib/Machines/Asynchronous Machine SI Units  RotorType=Wound  PresetModel=No  MechanicalLoad=Torque Tm  ShowDetailedParameters=on  ReferenceFrame=Rotor  Units=SI  MeasurementBus=off  NominalParameters=[ Ps Vs f ]  Stator=[ Rs , Lsi]  Rotor=[ Rr , Lsi]  Cage1=[ 0.022 0.226/377]  Cage2=[ 0.022 0.226/377]  Lm=Lm  Mechanical=[ J D 2 ]  PolePairs=2  InitialConditions=[1 0 0 0 0 0 0 0]  SimulateSaturation=off  Saturation=[14.03593122, 27.81365428, 53.79336849, 72.68890987, 97.98006896, 148.6815601, 215.7428561, 302.9841135, 420.4778367 ; 230, 322, 414, 460, 506, 552, 598, 644, 690]  LoadFlowParameters=1492000  TsPowergui=0  TsBlock=-1  IterativeModel=Trapezoidal non iterative  IterativeDiscreteModel=Trapezoidal non iterative  Pmec=0
  Constant2 : Constant  Value=0
  Constant3 : Constant  Value=Vbus_ref
  Control : Subsystem
  Control1 : Subsystem
  Deload method 1 : Subsystem
  Display{2..8,10..11,13} (10 alike) : Display
  Gain2 : Gain  Gain=1/(2*pi/60)
  Ground : powerlib/Elements/Ground  Commented=on  LConnTagsString=a
  MPPT & Deload method 2 : Subsystem
  Manual Switch : ManualSwitch  CurrentSetting=0
  Measurement of Power - Frequency : Subsystem
  Monitor DFIG : Subsystem
  Reativa ref : Constant  Value=0
  Scope : Scope  Commented=on
  Series RLC Branch : powerlib/Elements/Series RLC Branch  LConnTagsString=__new0  RConnTagsString=__new0  BranchType=C  Resistance=1  Inductance=1e-3  SetiL0=off  InitialCurrent=0  Capacitance=Cbus  Setx0=off  InitialVoltage=0  Measurements=Branch voltage
  Signal Builder : Subsystem  Tag=STV Subsys  LoadFcn=sigbuilder_block('load');  StartFcn=sigbuilder_block('start');  StopFcn=sigbuilder_block('stop');  ClipboardFcn=sigbuilder_block('clipboard');  mask(Sigbuilder block){tuvar=[0:10]}
      mask help: Simulink:masks:SigbuilderBlock_MD
      mask init:
      | if ~strcmp(get_param(bdroot(gcbh),'SimulationStatus'),'stopped') tuvar = sigbuilder_block('maskInit'); end
      settings: CopyFcn=sigbuilder_block('copy');  DeleteFcn=sigbuilder_block('delete');  ModelCloseFcn=sigbuilder_block('modelClose');  PreSaveFcn=sigbuilder_block('preSave');  PauseFcn=sigbuilder_block('pause');  ContinueFcn=sigbuilder_block('continue');  NameChangeFcn=sigbuilder_block('namechange');  OpenFcn=sigbuilder_block('open',[6 22.5 1012.5 455.25 ]);  CloseFcn=sigbuilder_block('close');
      mask Display: plot(0, 0, 100, 100,[2, 2, 32, 32, 2], [68, 8, 8, 68, 68],[32, 2], [38, 38], [32, 19, 2],[53, 60, 44], [32, 17, 17, 2],[16, 16, 31, 31]);txt = getActiveGroup(gcbh);text(2, 100, txt,'verticalAlignment', 'top');
  Subsystem : Subsystem
  Three-Phase Programmable Voltage Source : powerlib/Electrical Sources/Three-Phase Programmable Voltage Source  Commented=on  PositiveSequence="[Vs  0 f]"  VariationEntity=Frequency  VariationType=Table of time-amplitude pairs  VariationTypeAlt=Step  VariationStep=[-0.8]  VariationRate=10  VariationMagnitude=0.3  VariationFrequency=2  VariationTiming=[2 3]  VariationPhaseA=off  Amplitudes=[1 0.8 1.2 1.0]  TimeValues=[0 0.1 0.15 0.2]  HarmonicGeneration=off  HarmonicA=[3 0.2 -25 0]  HarmonicB=[2 0.15 35 2]  Timing="[0.05  3]"  BusType=swing  Pref=0  Qref=0  Qmin=-inf  Qmax=inf
  Three-Phase Series RLC Branch2 : powerlib/Elements/Three-Phase Series RLC Branch  LConnTagsString=A|B|C  RConnTagsString=A|B|C  BranchType=RL  Resistance=Rfilter*1.5  Inductance=Lfilter*0.8  Capacitance=0  Measurements=None
  Three-Phase Transformer (Two Windings) : powerlib/Elements/Three-Phase Transformer (Two Windings)  Winding1Connection=Y  Winding2Connection=Y  CoreType=Three single-phase transformers  SetSaturation=off  Hysteresis=off  DataFile='hysteresis'  SetInitialFlux=off  Measurements=None  UNITS=SI  NominalPower=[ Ps , f]  Winding1=[Vs 0 0]  Winding2=[Vs/u 0 0]  Rm=1.0805e+06  Lm=2866  L0=0.5  Saturation=[0 0;0.66653 1910.3;277.72 2419.7]  InitialFluxes=[1273.5 -1273.5 1114.3]  MoreParameters=off  BreakLoop=off  DataType=on  TransfoNumber=1
  Three-Phase V-I Measurement : powerlib/Measurements/Three-Phase V-I Measurement  VoltageMeasurement=phase-to-ground  SetLabelV=on  LabelV=Vs  Vpu=off  VpuLL=off  CurrentMeasurement=yes  SetLabelI=on  LabelI=Is  Ipu=off  Pbase=100e6  Vbase=500e3  OutputType=Complex  PhasorSimulation=off  PSBequivalent=0
  Three-Phase V-I Measurement1 : powerlib/Measurements/Three-Phase V-I Measurement  VoltageMeasurement=phase-to-phase  SetLabelV=on  LabelV=Vr  Vpu=off  VpuLL=off  CurrentMeasurement=yes  SetLabelI=on  LabelI=Ir  Ipu=off  Pbase=100e6  Vbase=500e3  OutputType=Complex  PhasorSimulation=off  PSBequivalent=0
  Three-Phase V-I Measurement2 : powerlib/Measurements/Three-Phase V-I Measurement  VoltageMeasurement=phase-to-ground  SetLabelV=on  LabelV=Vdfig  Vpu=off  VpuLL=off  CurrentMeasurement=yes  SetLabelI=on  LabelI=Idfig  Ipu=off  Pbase=100e6  Vbase=500e3  OutputType=Complex  PhasorSimulation=off  PSBequivalent=0
  Three-Phase V-I Measurement3 : powerlib/Measurements/Three-Phase V-I Measurement  VoltageMeasurement=phase-to-ground  SetLabelV=on  LabelV=Vgrid  Vpu=off  VpuLL=off  CurrentMeasurement=yes  SetLabelI=on  LabelI=Igrid  Ipu=off  Pbase=100e6  Vbase=500e3  OutputType=Complex  PhasorSimulation=off  PSBequivalent=0
  Universal Bridge : powerlib/Power Electronics/Universal Bridge  Arms=3  SnubberResistance=1e5  SnubberCapacitance=inf  Device=Ideal Switches  Ron=1e-3  Lon=0  ForwardVoltages="[  0  0  ]"  ForwardVoltage=0  GTOparameters=[ 10e-6 , 20e-6 ]  IGBTparameters=[ 1e-6 , 2e-6 ]  Measurements=None  Measurements_2=None  converterType=Rectifier
  Universal Bridge1 : powerlib/Power Electronics/Universal Bridge  Arms=3  SnubberResistance=1e5  SnubberCapacitance=inf  Device=Ideal Switches  Ron=1e-3  Lon=0  ForwardVoltages="[  0  0  ]"  ForwardVoltage=0  GTOparameters=[ 10e-6 , 20e-6 ]  IGBTparameters=[ 1e-6 , 2e-6 ]  Measurements=None  Measurements_2=None  converterType=Rectifier
  Voltage Measurement : powerlib/Measurements/Voltage Measurement  PhasorSimulation=off  OutputType=Complex  PSBequivalent=0
  Wind Trubine Model : Subsystem
  Wind speed (m/s) 1 : Constant  Value=11.5
  Zero-Order Hold{,1..2,4..8} (8 alike) : ZeroOrderHold  SampleTime=1/fsw
  beta1 : Constant  Value=beta
  ramp : Subsystem  Tag=STV Subsys  LoadFcn=sigbuilder_block('load');  StartFcn=sigbuilder_block('start');  StopFcn=sigbuilder_block('stop');  ClipboardFcn=sigbuilder_block('clipboard');  mask(Sigbuilder block){tuvar=[0:10]}
      mask help: Simulink:masks:SigbuilderBlock_MD
      mask init:
      | if ~strcmp(get_param(bdroot(gcbh),'SimulationStatus'),'stopped') tuvar = sigbuilder_block('maskInit'); end
      settings: CopyFcn=sigbuilder_block('copy');  DeleteFcn=sigbuilder_block('delete');  ModelCloseFcn=sigbuilder_block('modelClose');  PreSaveFcn=sigbuilder_block('preSave');  PauseFcn=sigbuilder_block('pause');  ContinueFcn=sigbuilder_block('continue');  NameChangeFcn=sigbuilder_block('namechange');  OpenFcn=sigbuilder_block('open',[6 22.5 1012.5 455.25 ]);  CloseFcn=sigbuilder_block('close');
      mask Display: plot(0, 0, 100, 100,[2, 2, 32, 32, 2], [68, 8, 8, 68, 68],[32, 2], [38, 38], [32, 19, 2],[53, 60, 44], [32, 17, 17, 2],[16, 16, 31, 31]);txt = getActiveGroup(gcbh);text(2, 100, txt,'verticalAlignment', 'top');
  ramp1 : Subsystem  Tag=STV Subsys  LoadFcn=sigbuilder_block('load');  StartFcn=sigbuilder_block('start');  StopFcn=sigbuilder_block('stop');  ClipboardFcn=sigbuilder_block('clipboard');  mask(Sigbuilder block){tuvar=[0:10]}
      mask help: Simulink:masks:SigbuilderBlock_MD
      mask init:
      | if ~strcmp(get_param(bdroot(gcbh),'SimulationStatus'),'stopped') tuvar = sigbuilder_block('maskInit'); end
      settings: CopyFcn=sigbuilder_block('copy');  DeleteFcn=sigbuilder_block('delete');  ModelCloseFcn=sigbuilder_block('modelClose');  PreSaveFcn=sigbuilder_block('preSave');  PauseFcn=sigbuilder_block('pause');  ContinueFcn=sigbuilder_block('continue');  NameChangeFcn=sigbuilder_block('namechange');  OpenFcn=sigbuilder_block('open',[0 22.5 1024.5 495.75 ]);  CloseFcn=sigbuilder_block('close');
      mask Display: plot(0, 0, 100, 100,[2, 2, 32, 32, 2], [68, 8, 8, 68, 68],[32, 2], [38, 38], [32, 19, 2],[53, 60, 44], [32, 17, 17, 2],[16, 16, 31, 31]);txt = getActiveGroup(gcbh);text(2, 100, txt,'verticalAlignment', 'top');
  A : PMIOPort  Port=1  Side=Right
  B : PMIOPort  Port=2  Side=Right
  C : PMIOPort  Port=3  Side=Right
  tag scope: GSC=global, Pot_backup=global, Pot_max_ref1=global, Pot_max_ref2=global, Pot_ref_deload1=global, Pot_ref_deload2=global, RSC=global, Tem_ref=global, Tm=global, Vbus=global, Wind_Speed=global
  wires:
  [Igrid] -> Zero-Order Hold5/1
  beta1/1 -> Wind Trubine Model/1(Pitch angle (°))
  Constant3/1 -> Zero-Order Hold7/1
  MPPT & Deload method 2/1(Tem_ref) -> [Tem_ref]
  Wind Trubine Model/1(Tm) -> [Tm]
  [Stator_Power] -> Display8/1
  [Tm] -> Asynchronous Machine SI Units/1
  MPPT & Deload method 2/2("Pot_max_ref ") -> [Pot_max_ref2]
  Reativa ref/1 -> Zero-Order Hold4/1
  [GSC] -> Universal Bridge1/1
  Wind Trubine Model/2(Pot_mechanical) -> Display2/1
  [omega_m] -> MPPT & Deload method 2/1(Omega_m)
  Control/1(PWM) -> [RSC]
  [tita_m] -> Zero-Order Hold/1
  [Rotor_Power] -> Display10/1
  [omega_m] -> Gain2/1
  [Vs] -> Zero-Order Hold2/1
  Asynchronous Machine SI Units/1 -> Subsystem/1(In1)
  Zero-Order Hold/1 -> Control/5(Theta_m (θm))
  Zero-Order Hold2/1 -> Control/4(Vabcs)
  Gain2/1 -> Display7/1
  Zero-Order Hold1/1 -> Control/3(iabcr)
  Constant2/1 -> Control/2(Q_ref)
  [Vbus] -> Zero-Order Hold8/1
  Zero-Order Hold7/1 -> Control1/1(Vbus_ref)
  [RSC] -> Universal Bridge/1
  [Ir] -> Zero-Order Hold1/1
  [Vs] -> Zero-Order Hold6/1
  Zero-Order Hold6/1 -> Control1/5("Vabcg ")
  Zero-Order Hold5/1 -> Control1/4(iabcg)
  Voltage Measurement/1 -> Display6/1, [Vbus]
  Zero-Order Hold4/1 -> Control1/3(Qg_ref)
  Control1/1(PWM) -> [GSC]
  Zero-Order Hold8/1 -> Control1/2(Vbus)
  Manual Switch/1 -> Scope/1, Display3/1, [Wind_Speed], Wind Trubine Model/2(Wind speed (m/s))
  Wind speed (m/s) 1/1 -> Manual Switch/1
  [Wind_Speed] -> Deload method 1/1(Wind speed (m/s))
  Deload method 1/1(P_deload) -> [Pot_ref_deload1]
  [Tem_ref] -> Control/1(Tem_ref)
  Deload method 1/2(P_Max) -> [Pot_max_ref1]
  Measurement of Power - Frequency/1(F (Hz)) -> Display11/1
  Measurement of Power - Frequency/3(Q (VAR)) -> Display13/1
  Measurement of Power - Frequency/2(P (W)) -> Display4/1
  Measurement of Power - Frequency/4(Angle (0)) -> Display5/1
  Deload method 1/3(P_backup) -> [Pot_backup]
  MPPT & Deload method 2/3("Pot_ref_deload2 ") -> [Pot_ref_deload2]
  ramp1/1(Signal 1) -> Manual Switch/2
  connections:
  Three-Phase V-I Measurement/RConn2 -- Three-Phase V-I Measurement2/LConn2 -- Three-Phase V-I Measurement3/RConn2
  Three-Phase V-I Measurement2/RConn1 -- A/RConn1 -- Three-Phase Programmable Voltage Source/RConn1
  Voltage Measurement/LConn2 -- Universal Bridge1/RConn2 -- Universal Bridge/RConn2 -- Series RLC Branch/RConn1
  Universal Bridge1/RConn1 -- Voltage Measurement/LConn1 -- Universal Bridge/RConn1 -- Series RLC Branch/LConn1
  Three-Phase V-I Measurement/RConn3 -- Three-Phase V-I Measurement2/LConn3 -- Three-Phase V-I Measurement3/RConn3
  Three-Phase Transformer (Two Windings)/LConn2 -- Asynchronous Machine SI Units/RConn2
  Three-Phase Transformer (Two Windings)/LConn3 -- Asynchronous Machine SI Units/RConn3
  Three-Phase V-I Measurement1/LConn1 -- Universal Bridge/LConn1
  Three-Phase V-I Measurement/LConn1 -- Asynchronous Machine SI Units/LConn1
  Three-Phase Transformer (Two Windings)/LConn1 -- Asynchronous Machine SI Units/RConn1
  Three-Phase V-I Measurement/LConn3 -- Asynchronous Machine SI Units/LConn3
  Three-Phase Transformer (Two Windings)/RConn3 -- Three-Phase V-I Measurement1/RConn3
  Three-Phase V-I Measurement1/LConn3 -- Universal Bridge/LConn3
  Three-Phase V-I Measurement1/LConn2 -- Universal Bridge/LConn2
  Three-Phase Transformer (Two Windings)/RConn2 -- Three-Phase V-I Measurement1/RConn2
  Three-Phase V-I Measurement/LConn2 -- Asynchronous Machine SI Units/LConn2
  Three-Phase Transformer (Two Windings)/RConn1 -- Three-Phase V-I Measurement1/RConn1
  Ground/LConn1 -- Three-Phase Programmable Voltage Source/LConn1
  Three-Phase V-I Measurement/RConn1 -- Three-Phase V-I Measurement2/LConn1 -- Three-Phase V-I Measurement3/RConn1
  Three-Phase Programmable Voltage Source/RConn3 -- Three-Phase V-I Measurement2/RConn3 -- C/RConn1
  Three-Phase V-I Measurement2/RConn2 -- B/RConn1 -- Three-Phase Programmable Voltage Source/RConn2
  Three-Phase Series RLC Branch2/RConn2 -- Three-Phase V-I Measurement3/LConn2
  Three-Phase Series RLC Branch2/RConn3 -- Three-Phase V-I Measurement3/LConn3
  Universal Bridge1/LConn1 -- Three-Phase Series RLC Branch2/LConn1
  Universal Bridge1/LConn2 -- Three-Phase Series RLC Branch2/LConn2
  Universal Bridge1/LConn3 -- Three-Phase Series RLC Branch2/LConn3
  Three-Phase Series RLC Branch2/RConn1 -- Three-Phase V-I Measurement3/LConn1

== system DFIG_BESS_In_power_LFnetwork_5bus/Frequency Load ==
  PLL (3ph)1 : powerlib_meascontrol/PLL/PLL (3ph)  Fmin=45  Par_Init=[0, f]  ParK=[180, 3200, 1]  TcD=1e-4  MaxRateChangeFreq=12  FilterCutOffFreq=25  Ts=0  AGC=on
  tag scope: f_plant=global
  wires:
  [Vabc_h_plant] -> PLL (3ph)1/1
  PLL (3ph)1/1 -> [f_plant]

== system DFIG_BESS_In_power_LFnetwork_5bus/Frequency DFIG - BESS ==
  PLL (3ph)1 : powerlib_meascontrol/PLL/PLL (3ph)  Fmin=45  Par_Init=[0, f]  ParK=[180, 3200, 1]  TcD=1e-4  MaxRateChangeFreq=12  FilterCutOffFreq=25  Ts=0  AGC=on
  tag scope: f_dfig_bess=global
  wires:
  PLL (3ph)1/1 -> [f_dfig_bess]
  [V_ac_g] -> PLL (3ph)1/1

== system DFIG_BESS_In_power_LFnetwork_5bus/Load N°1 49MW 12Mvar ==
  note: Consumer Load
  3-Phase Breaker : powerlib/Elements/Three-Phase Breaker  Commented=on  InitialState=open  SwitchA=on  SwitchB=on  SwitchC=on  SwitchTimes=[4]  External=off  BreakerResistance=0.001  SnubberResistance=1e6  SnubberCapacitance=inf  Measurements=None
      settings: AttributesFormatString=\n
  Load : powerlib/Measurements/Three-Phase V-I Measurement  VoltageMeasurement=no  SetLabelV=on  LabelV=Vabc_Load_B2  Vpu=off  VpuLL=off  CurrentMeasurement=no  SetLabelI=on  LabelI=Iabc_Load_B2  Ipu=off  Pbase=25e3  Vbase=480  OutputType=Magnitude  PhasorSimulation=off  PSBequivalent=0
  Main Load 10MW : powerlib/Elements/Three-Phase Parallel RLC Load  LConnTagsString=A|B|C  Configuration=Y (grounded)  NominalVoltage=33e+03  Vabc=[1e3 1e3 1e3]  Vabcp=[1e3 1e3 1e3]  NominalFrequency=60  UnbalancedPower=off  ActivePower=49e+06  InductivePower=12e+06  CapacitivePower=0  Pabc=[10e3 9e3 11e3]  QLabc=[100 90 110]  QCabc=[100 90 110]  Pabcp=[10e3 9e3 11e3]  QLabcp=[100 90 110]  QCabcp=[100 90 110]  Measurements=None  LoadType=constant Z
  Main Load 5M : powerlib/Elements/Three-Phase Parallel RLC Load  Commented=on  LConnTagsString=A|B|C  Configuration=Y (grounded)  NominalVoltage=33e+03  Vabc=[1e3 1e3 1e3]  Vabcp=[1e3 1e3 1e3]  NominalFrequency=60  UnbalancedPower=off  ActivePower=5e+06  InductivePower=0  CapacitivePower=0  Pabc=[10e3 9e3 11e3]  QLabc=[100 90 110]  QCabc=[100 90 110]  Pabcp=[10e3 9e3 11e3]  QLabcp=[100 90 110]  QCabcp=[100 90 110]  Measurements=None  LoadType=constant Z
  PLL (3ph)1 : powerlib_meascontrol/PLL/PLL (3ph)  Commented=on  Fmin=45  Par_Init=[0, f]  ParK=[180, 3200, 1]  TcD=1e-4  MaxRateChangeFreq=12  FilterCutOffFreq=25  Ts=0  AGC=on
  "Power (3ph, Instantaneous)1" : powerlib_meascontrol/Measurements/Power (3ph, Instantaneous)  Commented=on
      settings: SourceProductName=Simscape Power Systems
  Scope : Scope  Commented=on
  Vbus vcc1 : From  Commented=on  GotoTag=Iabc_Load_B2  TagVisibility=global
  Vbus vcc2 : From  Commented=on  GotoTag=Vabc_Load_B2  TagVisibility=global
  A : PMIOPort  Port=1  Side=Right
  B : PMIOPort  Port=2  Side=Right
  C : PMIOPort  Port=3  Side=Right
  wires:
  "Power (3ph, Instantaneous)1"/1 -> Scope/1
  Vbus vcc2/1 -> "Power (3ph, Instantaneous)1"/1, PLL (3ph)1/1
  Vbus vcc1/1 -> "Power (3ph, Instantaneous)1"/2
  connections:
  C/RConn1 -- Load/LConn3
  B/RConn1 -- Load/LConn2
  A/RConn1 -- Load/LConn1
  3-Phase Breaker/RConn3 -- Main Load 5M/LConn3
  3-Phase Breaker/RConn1 -- Main Load 5M/LConn1
  3-Phase Breaker/RConn2 -- Main Load 5M/LConn2
  Load/RConn1 -- 3-Phase Breaker/LConn1 -- Main Load 10MW/LConn1
  Load/RConn3 -- 3-Phase Breaker/LConn3 -- Main Load 10MW/LConn3
  Load/RConn2 -- 3-Phase Breaker/LConn2 -- Main Load 10MW/LConn2
